simulink model "sin_gen_my_ref"  (R2015b)
settings: Solver=ode45  StartTime=0.0  StopTime=1e-6  RelTol=1e-3
libraries: simulink x2, commutil2 x2
settings Model: Creator=Admin  LastModifiedBy=alexe
settings DataIOCC: SaveFormat=Array  SignalLoggingSaveFormat=ModelDataLogs
settings OptimizationCC: ExpressionDepthLimit=2147483647
settings DebuggingCC: UnderspecifiedInitializationDetection=Classic  MergeDetectMultiDrivingBlocksExec=none  SolverPrmCheckMsg=warning  FcnCallInpInsideContextMsg=UseLocalSettings  StateNameClashWarn=warning
settings HardwareCC: ProdBitPerPointer=32  ProdLargestAtomicFloat=None  ProdIntDivRoundTo=Undefined  ProdEndianess=Unspecified  ProdWordSize=32  ProdHWDeviceType=32-bit Generic
settings GRTTargetCC: GeneratePreprocessorConditionals=Disable all  CombineOutputUpdateFcns=off  GRTInterface=on
settings ConfigComp: CovModelRefEnable=Off

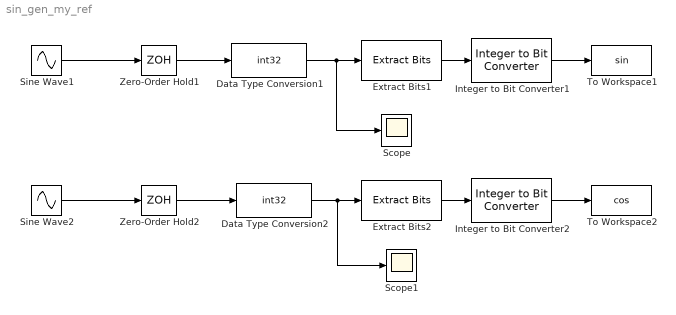
== system sin_gen_my_ref ==
  Data Type Conversion1 : DataTypeConversion  OutDataTypeStr=int32  RndMeth=Round  SampleTime=1/4096e6
  Data Type Conversion2 : DataTypeConversion  OutDataTypeStr=int32  RndMeth=Round  SampleTime=1/4096e6
  Extract Bits1 : simulink/Logic and Bit Operations/Extract Bits  bitsToExtract=Range of bits  numBits=8  bitIdxRange=[0 17]  outScalingMode=Preserve fixed-point scaling
  Extract Bits2 : simulink/Logic and Bit Operations/Extract Bits  bitsToExtract=Range of bits  numBits=8  bitIdxRange=[0 17]  outScalingMode=Preserve fixed-point scaling
  Integer to Bit Converter1 : commutil2/Integer to Bit Converter  nbits=18  signedInputValues=Signed  bitOrder=MSB first  outDtype=Inherit via internal rule
  Integer to Bit Converter2 : commutil2/Integer to Bit Converter  nbits=18  signedInputValues=Signed  bitOrder=MSB first  outDtype=Inherit via internal rule
  Scope : Scope
  Scope1 : Scope
  Sine Wave1 : Sin  Amplitude=-131071  Frequency=2*pi*1e6  SampleTime=0
  Sine Wave2 : Sin  Amplitude=131071  Frequency=2*pi*1e6  Phase=pi/2  SampleTime=0
  To Workspace1 : ToWorkspace  VariableName=sin  SampleTime=1/4096e6
  To Workspace2 : ToWorkspace  VariableName=cos  SampleTime=1/4096e6
  Zero-Order Hold1 : ZeroOrderHold  SampleTime=1/4096e6
  Zero-Order Hold2 : ZeroOrderHold  SampleTime=1/4096e6
  wires:
  Zero-Order Hold1/1 -> Data Type Conversion1/1
  Integer to Bit Converter1/1 -> To Workspace1/1
  Data Type Conversion1/1 -> Extract Bits1/1, Scope/1
  Extract Bits1/1 -> Integer to Bit Converter1/1
  Sine Wave1/1 -> Zero-Order Hold1/1
  Zero-Order Hold2/1 -> Data Type Conversion2/1
  Integer to Bit Converter2/1 -> To Workspace2/1
  Data Type Conversion2/1 -> Scope1/1, Extract Bits2/1
  Extract Bits2/1 -> Integer to Bit Converter2/1
  Sine Wave2/1 -> Zero-Order Hold2/1
